simulink model "Model"  (R2020b)
settings: Solver=VariableStepAuto  StartTime=0.0  StopTime=100  MaxStep=0.1  RelTol=1e-3
model workspace (MAT data in the model file):
  B = 1000
  K = 16000
  K2 = 200000
  M1 = 300
  M2 = 20
settings Model: DataDictionary=Data.sldd  OrderedModelArguments=off  Creator=user  LastModifiedBy=user
settings DataIOCC: ExternalInput=[t, road]  LoadExternalInput=on

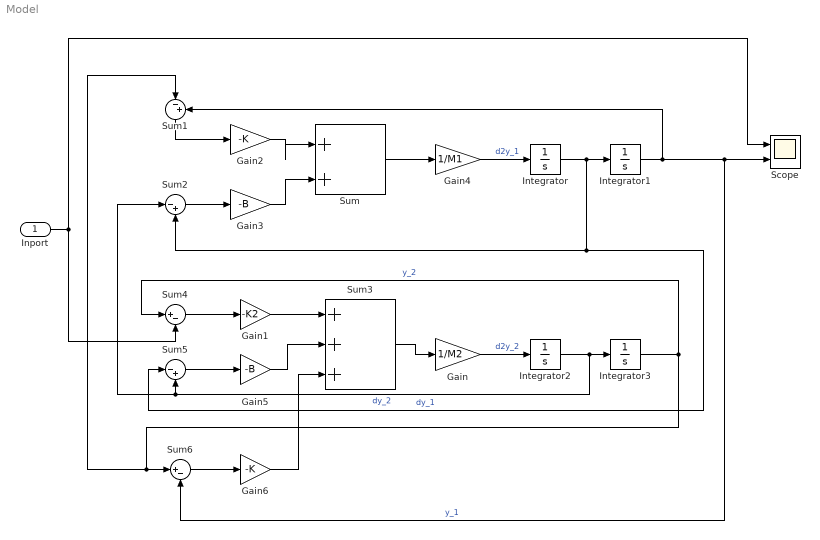
== system Model ==
  Inport : Inport
  Gain : Gain  Gain=1/M2
  Gain1 : Gain  Gain=-K2
  Gain2 : Gain  Gain=-K
  Gain3 : Gain  Gain=-B
  Gain4 : Gain  Gain=1/M1
  Gain5 : Gain  Gain=-B
  Gain6 : Gain  Gain=-K
  Integrator{,1..3} (4 alike) : Integrator
  Scope : Scope  NumInputPorts=2
  Sum : Sum  Inputs=|++
  Sum1 : Sum  Inputs=|-+
  Sum2 : Sum  Inputs=|-+
  Sum3 : Sum  Inputs=+|++
  Sum4 : Sum  Inputs=|+-
  Sum5 : Sum  Inputs=|-+
  Sum6 : Sum  Inputs=|+-
  wires:
  Integrator/1 -> Sum5/1, Sum2/2, Integrator1/1  "dy_1"
  Sum/1 -> Gain4/1
  Gain4/1 -> Integrator/1  "d2y_1"
  Sum1/1 -> Gain2/1
  Sum2/1 -> Gain3/1
  Integrator1/1 -> Sum1/2, Sum6/2, Scope/2  "y_1"
  Gain3/1 -> Sum/2
  Gain2/1 -> Sum/1
  Sum3/1 -> Gain/1
  Gain/1 -> Integrator2/1  "d2y_2"
  Integrator2/1 -> Sum2/1, Sum5/2, Integrator3/1  "dy_2"
  Integrator3/1 -> Sum6/1, Sum1/1, Sum4/1  "y_2"
  Sum4/1 -> Gain1/1
  Gain1/1 -> Sum3/1
  Sum5/1 -> Gain5/1
  Gain5/1 -> Sum3/2
  Sum6/1 -> Gain6/1
  Gain6/1 -> Sum3/3
  Inport/1 -> Sum4/2, Scope/1
